simulink model "Model_PI_lambdaD"  (Simulink 9.2)
settings: Solver=FixedStepAuto  StartTime=0.0  StopTime=20  FixedStep=T_s  RelTol=1e-3  EnableMultiTasking=on
values from neighbouring files (symbols this model uses):
  disturb_step_time = handles.disTime    [GUI_Comparison1.m]    (also in GUI_Comparison2.m; GUI_Main.m = str2double(get(handles.edit_disTime,   'string')); function_PI_lambdaD.m = 100; programEx6PILamD.m = 40)
  disturb_step_value = handles.disValue    [GUI_Comparison1.m]    (also in GUI_Comparison2.m; GUI_Main.m = str2double(get(handles.edit_disValue,  'string')); function_PI_lambdaD.m = 0.5; programEx6PILamD.m = 0.5)
  kd = kd_array(j)    [function_PI_lambdaD.m]    (also in programEx6PILamD.m = 6.82)
  ki = 230.216    [programEx6PILamD.m]
  kp = 97.7464    [programEx6PILamD.m]
  L = handles.L    [GUI_Comparison1.m]    (also in GUI_Comparison2.m; GUI_Main.m; function_PI_lambdaD.m = delay; irid_fod.m = 200)
  lambda = mu * r2    [GUI_Main.m]    (also in function_FOPID.m; function_FOPID_para.m; function_PI_lambdaD.m = rsc_lambda(j,k); programEx6PILamD.m = 1.49)
  step_value = handles.stepValue    [GUI_Comparison1.m]    (also in GUI_Comparison2.m; GUI_Main.m = str2double(get(handles.edit_stepValue, 'string')); programEx6PILamD.m = 1)
libraries: cstblocks x3, powerlib x1
settings Model: Creator=Li Chuang  LastModifiedBy=18764
settings SolverCC: AlgebraicLoopSolver=LineSearch
settings OptimizationCC: InitFltsAndDblsToZero=on
settings DebuggingCC: SaveWithParameterizedLinksMsg=none  SignalResolutionControl=TryResolveAllWithWarning  SolverPrmCheckMsg=warning  MultiTaskDSMMsg=warning  MultiTaskCondExecSysMsg=none  FcnCallInpInsideContextMsg=error  AllowSymbolicDim=off  StateNameClashWarn=none
settings GRTTargetCC: TargetFcnLib=ansi_tfl_tmw.mat  GeneratePreprocessorConditionals=Use local settings

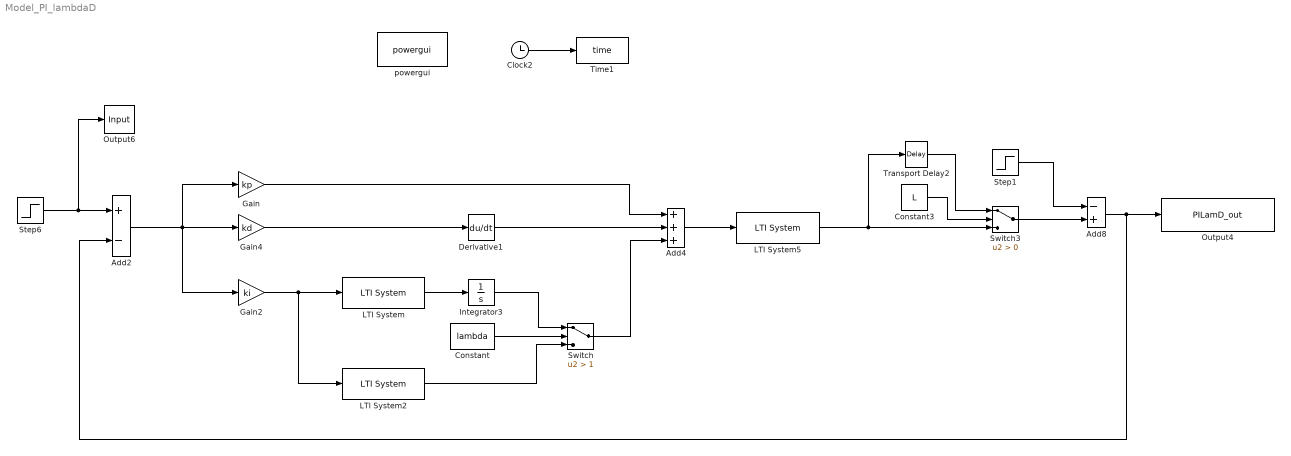
== system Model_PI_lambdaD ==
  Add2 : Sum  Inputs=+-  SaturateOnIntegerOverflow=on  OutDataTypeStr=Inherit: Same as first input
  Add4 : Sum  Inputs=+++  SaturateOnIntegerOverflow=on  OutDataTypeStr=Inherit: Same as first input
  Add8 : Sum  Inputs=-+  SaturateOnIntegerOverflow=on  OutDataTypeStr=Inherit: Same as first input
  Clock2 : Clock
      settings: Decimation=100
  Constant : Constant  Value=lambda
  Constant3 : Constant  Value=L
  Derivative1 : Derivative
  Gain : Gain  Gain=kp
  Gain2 : Gain  Gain=ki
  Gain4 : Gain  Gain=kd
  Integrator3 : Integrator
  LTI System : cstblocks/LTI System  sys=dfod  IC=[]
  LTI System2 : cstblocks/LTI System  sys=dfod  IC=[]
  LTI System5 : cstblocks/LTI System  sys=Gp  IC=[]
  Output4 : ToWorkspace  VariableName=PILamD_out  SampleTime=-1
  Output6 : ToWorkspace  VariableName=Input  SampleTime=-1
  Step1 : Step  Time=disturb_step_time  After=disturb_step_value
  Step6 : Step  Time=0  After=step_value
  Switch : Switch  Criteria=u2 > Threshold  Threshold=1
  Switch3 : Switch  Criteria=u2 > Threshold
  Time1 : ToWorkspace  VariableName=time  SampleTime=-1
  Transport Delay2 : TransportDelay  DelayTime=L
  powergui : powerlib/powergui  Priority=1  SimulationMode=Discrete  SampleTime=50e-6  frequency=60  Iterations=50  frequencyindice=60  Pbase=100e6  ErrMax=1e-4  UnitsV=kV  UnitsW=MW  buscounter=0  FunctionMessages=off  echomessages=off  EnableUseOfTLC=off  CurrentSourceSwitches=off  DisableSnubberDevices=off  DisableRonSwitches=off  DisableVfSwitches=off  DisplayEquations=off  SolverType=Tustin/Backward Euler (TBE)  Interpol=off  ExternalGateDelay=off  methode=off  Ts=100  x0status=blocks  SPID=off  SwTol=0  HookPort=off  RestoreLinks=warning  ResistiveCurrentMeasurement=off  Frange=[0:2:500]  Ylog=off  Xlog=on  ShowGrid=off  save=off  variable=ZData  structure=0  ZoomFFT=off  StartTime=0.0  cycles=1  DisplayStyle=1  fundamental=60  FreqAxis=off  MaxFrequency=1000  frequencyindicesteady=1  RmsSteady=1  display=off
  wires:
  Add4/1 -> LTI System5/1
  Clock2/1 -> Time1/1
  Add8/1 -> Output4/1, Add2/2
  Transport Delay2/1 -> Switch3/1
  Constant3/1 -> Switch3/2
  LTI System5/1 -> Switch3/3, Transport Delay2/1
  Switch3/1 -> Add8/2
  Step6/1 -> Output6/1, Add2/1
  Step1/1 -> Add8/1
  Gain4/1 -> Derivative1/1
  Derivative1/1 -> Add4/2
  Gain/1 -> Add4/1
  Switch/1 -> Add4/3
  Add2/1 -> Gain2/1, Gain4/1, Gain/1
  LTI System2/1 -> Switch/3
  Constant/1 -> Switch/2
  Gain2/1 -> LTI System2/1, LTI System/1
  Integrator3/1 -> Switch/1
  LTI System/1 -> Integrator3/1
